simulink model "sampleModel1846"  (R2023a)
settings: Solver=VariableStepAuto  StartTime=0.0  StopTime=10.0  RelTol=1e-3
libraries: hdlsllib x6, simulink x3
settings Model: Creator=user1  LastModifiedBy=user1

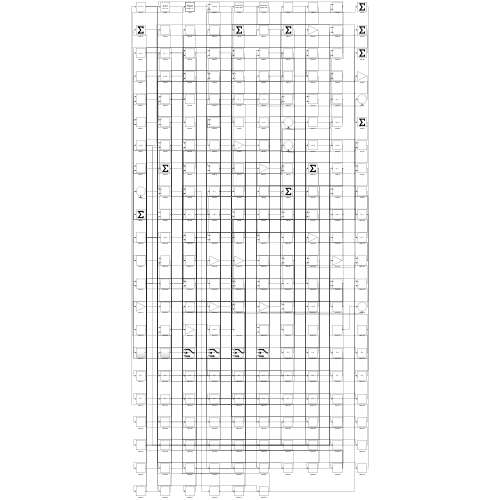
[thumbnail: Simulink's stored preview of the top-level diagram]
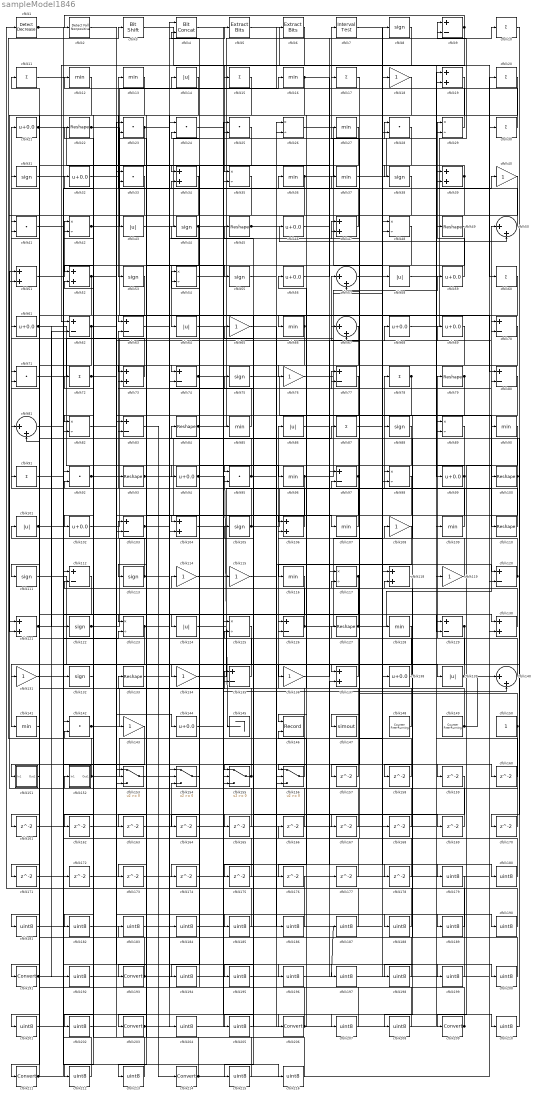
== system sampleModel1846 ==
  cfblk1 : simulink/Logic and Bit Operations/Detect Decrease  vinit=0.0  OutDataTypeStr=boolean
      settings: LibrarySourceBlock=|
      | hdlsllib/Logic and Bit
      | Operations/Detect
      | Decrease
  cfblk{10..11,15,17,20,30,60,72,78,87,91} (11 alike) : Sum  Inputs=+
  cfblk{22,45,49,79,84,93,100,110,127,133} (10 alike) : Reshape
  cfblk{14,43,58,64,86,101,124,139} (8 alike) : Abs  SaturateOnIntegerOverflow=off
  cfblk{21,32,46,56,59,61,68..69,94,99,102,138,144} (13 alike) : Bias  Bias=0.0  SaturateOnIntegerOverflow=off
  cfblk{9,62..63,70,74,77,80,83,97,103,112,120,126,129,135} (15 alike) : Sum  Inputs=+-
  cfblk{19,34,39,47,51..52,73,104,106,118,121,130,137} (13 alike) : Sum
  cfblk{8,31,38,44,53,55,75,88,105,111,113,122,132} (13 alike) : Signum
  cfblk{12..13,16,27,36..37,66,85,90,96,107,109,116,128,141} (15 alike) : MinMax
  cfblk{18,40,65,76,108,114..115,119,131,134,136,143} (12 alike) : Gain
  cfblk{26,29,35,42,48,54,82,89,98,117,123,125} (12 alike) : Product  Inputs=*/  RndMeth=Zero  SaturateOnIntegerOverflow=on
  cfblk{50,57,67,81,140} (5 alike) : Sum  Inputs=|++
  cfblk{23..25,28,33,41,71,92,95,142} (10 alike) : DotProduct  OutDataTypeStr=Inherit: Inherit via internal rule
  cfblk145 : Terminator
  cfblk146 : Record  FileSettingsInternal="{\"entries\":[{\"content\":{\"excelSettings\":{\"content\":{},\"type\":\"Streamout.ExcelSettings\"}},\"type\":\"Streamout.FileSettingStorage\",\"uuid\":\"\"}],\"packageUris\":[\"http:\\/\\/schema.mathworks.com\\/mf0\\/streamout_blocks\\/R2020a\"],\"version\":\"1.0\"}"  Layout=[1 1]  SignalsInternal="{\"entries\":[{\"content\":{\"signals\":[{\"content\":{\"blockPath\":[],\"dimensions\":[1],\"domain\":\"\",\"lineColor\":\"#a2142f\",\"plots\":[1],\"port\":1,\"signalID\":4512,\"signalName\":\"XY Graph:1\"},\"type\":\"RecordBlkView.Signal\",\"uuid\":\"\"},{\"content\":{\"blockPath\":[],\"dimensions\":[1],\"domain\":\"\",\"lineColor\":\"#139fff\",\"plots\":[1],\"port\":2,\"signalID\":4515,\"signalName\":\"XY Graph:2\"},\"type\":\"RecordBlkView.Signal\",\"uuid\":\"\"}]},\"type\":\"RecordBlkView.InputSignals\",\"uuid\":\"\"}],\"packageUris\":[\"http:\\/\\/schema.mathworks.com\\/mf0\\/streamout_blocks\\/R2020a\"],\"version\":\"1.0\"}"  VisualizationBindings="{\"xyplotplugin\":{\"info\":[{\"series\":[{\"bindingParametersList\":[{\"parameter\":\"X-Axis\",\"signalID\":4512,\"signalName\":\"XY Graph:1\"},{\"parameter\":\"Y-Axis\",\"signalID\":4515,\"signalName\":\"XY Graph:2\"}],\"seriesID\":51865}],\"subplotID\":1}]}}"  CompatibilityTag=XY  st=-1
  cfblk147 : ToWorkspace  VariableName=simout  SaveFormat=Timeseries  SampleTime=-1
  cfblk148 : hdlsllib/Sources/Counter Free-Running  NumBits=16  tsamp=-1
  cfblk149 : hdlsllib/Sources/Counter Free-Running  NumBits=16  tsamp=-1
  cfblk150 : Constant  SampleTime=-1
  cfblk151 : Subsystem
      settings: LibrarySourceBlock=|
      | hdlsllib/Ports &
      | Subsystems/Subsystem
  cfblk152 : Subsystem
      settings: LibrarySourceBlock=|
      | hdlsllib/Ports &
      | Subsystems/Subsystem
  cfblk{153..156} (4 alike) : Switch  SaturateOnIntegerOverflow=off  InputSameDT=off
  cfblk{157..178} (22 alike) : Delay  SampleTime=1
  cfblk{179..190,192,194..202,204..205,207..208,210,212..213,215..216} (31 alike) : DataTypeConversion  OutDataTypeStr=uint8  SaturateOnIntegerOverflow=off  RndMeth=Floor
  cfblk{191,193,203,206,209,211,214} (7 alike) : DataTypeConversion  SaturateOnIntegerOverflow=off  RndMeth=Floor
  cfblk2 : hdlsllib/Logic and Bit Operations/Detect Fall Nonpositive  vinit=0  OutDataTypeStr=boolean
  cfblk3 : hdlsllib/Logic and Bit Operations/Bit Shift  mode=Shift Left Logical  N=0
  cfblk4 : hdlsllib/Logic and Bit Operations/Bit Concat  numInputs=2
  cfblk5 : simulink/Logic and Bit Operations/Extract Bits  bitsToExtract=Upper half  numBits=8  bitIdxRange=[0 7]  outScalingMode=Preserve fixed-point scaling
      settings: LibrarySourceBlock=|
      | hdlsllib/Logic and Bit
      | Operations/Extract Bits
  cfblk6 : simulink/Logic and Bit Operations/Extract Bits  bitsToExtract=Upper half  numBits=8  bitIdxRange=[0 7]  outScalingMode=Preserve fixed-point scaling
      settings: LibrarySourceBlock=|
      | hdlsllib/Logic and Bit
      | Operations/Extract Bits
  cfblk7 : hdlsllib/Logic and Bit Operations/Interval Test  IntervalClosedRight=on  uplimit=0.5  IntervalClosedLeft=on  lowlimit=-0.5  OutDataTypeStr=boolean
  wires:
  cfblk29/1 -> cfblk12/1
  cfblk93/1 -> cfblk107/1, cfblk26/1, cfblk173/1
  cfblk121/1 -> cfblk62/2, cfblk123/2, cfblk199/1
  cfblk68/1 -> cfblk9/1
  cfblk127/1 -> cfblk50/1, cfblk45/1
  cfblk8/1 -> cfblk62/1
  cfblk66/1 -> cfblk63/1, cfblk155/1, cfblk123/1
  cfblk156/1 -> cfblk86/1
  cfblk51/1 -> cfblk42/1
  cfblk111/1 -> cfblk136/1
  cfblk99/1 -> cfblk95/1, cfblk155/2
  cfblk76/1 -> cfblk69/1
  cfblk130/1 -> cfblk32/1
  cfblk32/1 -> cfblk16/1
  cfblk10/1 -> cfblk137/1
  cfblk37/1 -> cfblk29/1
  cfblk47/1 -> cfblk13/1
  cfblk5/1 -> cfblk60/1
  cfblk61/1 -> cfblk96/1, cfblk192/1
  cfblk84/1 -> cfblk10/1, cfblk196/1
  cfblk148/1 -> cfblk126/1
  cfblk94/1 -> cfblk145/1, cfblk140/2
  cfblk140/1 -> cfblk79/1
  cfblk9/1 -> cfblk2/1, cfblk15/1
  cfblk45/1 -> cfblk50/2, cfblk37/1
  cfblk4/1 -> cfblk206/1
  cfblk123/1 -> cfblk141/1, cfblk167/1
  cfblk73/1 -> cfblk21/1
  cfblk91/1 -> cfblk36/1
  cfblk34/1 -> cfblk52/1
  cfblk42/1 -> cfblk6/1, cfblk197/1
  cfblk44/1 -> cfblk74/2, cfblk189/1, cfblk213/1
  cfblk69/1 -> cfblk147/1
  cfblk31/1 -> cfblk55/1
  cfblk27/1 -> cfblk82/1
  cfblk152/1(Out1) -> cfblk3/1, cfblk8/1
  cfblk106/1 -> cfblk63/2
  cfblk139/1 -> cfblk56/1, cfblk67/1
  cfblk134/1 -> cfblk70/1
  cfblk96/1 -> cfblk59/1, cfblk174/1
  cfblk92/1 -> cfblk57/1, cfblk94/1
  cfblk26/1 -> cfblk128/1
  cfblk75/1 -> cfblk110/1
  cfblk102/1 -> cfblk46/1
  cfblk56/1 -> cfblk9/2
  cfblk22/1 -> cfblk80/1, cfblk34/1
  cfblk110/1 -> cfblk41/1
  cfblk1/1 -> cfblk130/1, cfblk135/2, cfblk153/2
  cfblk107/1 -> cfblk81/1
  cfblk141/1 -> cfblk11/1
  cfblk50/1 -> cfblk29/2
  cfblk124/1 -> cfblk78/1
  cfblk38/1 -> cfblk76/1
  cfblk151/1(Out1) -> cfblk71/1
  cfblk55/1 -> cfblk40/1
  cfblk72/1 -> cfblk102/1, cfblk68/1
  cfblk18/1 -> cfblk193/1
  cfblk49/1 -> cfblk64/1
  cfblk14/1 -> cfblk53/1
  cfblk125/1 -> cfblk203/1
  cfblk79/1 -> cfblk116/1, cfblk208/1
  cfblk105/1 -> cfblk30/1, cfblk22/1
  cfblk149/1 -> cfblk140/1, cfblk126/2
  cfblk144/1 -> cfblk95/2
  cfblk3/1 -> cfblk99/1
  cfblk113/1 -> cfblk41/2, cfblk77/1
  cfblk6/1 -> cfblk35/1
  cfblk71/1 -> cfblk43/1
  cfblk112/1 -> cfblk211/1
  cfblk20/1 -> cfblk191/1
  cfblk43/1 -> cfblk7/1
  cfblk23/1 -> cfblk5/1, cfblk151/1(In1)
  cfblk132/1 -> cfblk72/1
  cfblk16/1 -> cfblk97/1, cfblk104/2
  cfblk35/1 -> cfblk73/1
  cfblk155/1 -> cfblk103/1, cfblk81/2
  cfblk58/1 -> cfblk100/1
  cfblk154/1 -> cfblk84/1
  cfblk59/1 -> cfblk39/1
  cfblk104/1 -> cfblk98/1
  cfblk64/1 -> cfblk28/1
  cfblk150/1 -> cfblk152/1(In1), cfblk47/2
  cfblk119/1 -> cfblk108/1
  cfblk39/1 -> cfblk38/1, cfblk155/3
  cfblk135/1 -> cfblk93/1
  cfblk153/1 -> cfblk87/1
  cfblk120/1 -> cfblk88/1, cfblk106/2
  cfblk25/1 -> cfblk104/1
  cfblk109/1 -> cfblk27/1
  cfblk138/1 -> cfblk71/2
  cfblk95/1 -> cfblk120/1, cfblk52/2
  cfblk100/1 -> cfblk31/1, cfblk113/1, cfblk170/1
  cfblk62/1 -> cfblk144/1, cfblk111/1
  cfblk142/1 -> cfblk115/1, cfblk135/1
  cfblk88/1 -> cfblk134/1
  cfblk78/1 -> cfblk103/2, cfblk153/3
  cfblk126/1 -> cfblk48/1, cfblk54/1
  cfblk28/1 -> cfblk48/2
  cfblk129/1 -> cfblk146/1, cfblk202/1
  cfblk41/1 -> cfblk39/2
  cfblk122/1 -> cfblk25/2, cfblk85/1
  cfblk52/1 -> cfblk106/1, cfblk161/1
  cfblk90/1 -> cfblk209/1
  cfblk101/1 -> cfblk139/1, cfblk34/2, cfblk210/1, cfblk216/1
  cfblk21/1 -> cfblk117/1, cfblk207/1
  cfblk53/1 -> cfblk82/2
  cfblk85/1 -> cfblk23/2
  cfblk30/1 -> cfblk17/1
  cfblk131/1 -> cfblk132/1
  cfblk137/1 -> cfblk127/1
  cfblk136/1 -> cfblk70/2
  cfblk98/1 -> cfblk154/2
  cfblk36/1 -> cfblk19/1, cfblk121/2
  cfblk12/1 -> cfblk51/2
  cfblk97/1 -> cfblk44/1, cfblk156/2
  cfblk115/1 -> cfblk80/2
  cfblk48/1 -> cfblk156/1
  cfblk74/1 -> cfblk28/2, cfblk124/1, cfblk54/2
  cfblk19/1 -> cfblk66/1
  cfblk116/1 -> cfblk131/1
  cfblk83/1 -> cfblk214/1
  cfblk57/1 -> cfblk129/2
  cfblk103/1 -> cfblk47/1, cfblk77/2, cfblk163/1
  cfblk40/1 -> cfblk74/1
  cfblk117/1 -> cfblk67/2, cfblk212/1
  cfblk17/1 -> cfblk157/1
  cfblk157/1 -> cfblk25/1
  cfblk80/1 -> cfblk158/1
  cfblk158/1 -> cfblk57/2
  cfblk82/1 -> cfblk159/1
  cfblk86/1 -> cfblk160/1
  cfblk160/1 -> cfblk129/1
  cfblk161/1 -> cfblk154/3
  cfblk13/1 -> cfblk162/1
  cfblk162/1 -> cfblk98/2
  cfblk163/1 -> cfblk19/2
  cfblk77/1 -> cfblk164/1
  cfblk81/1 -> cfblk165/1
  cfblk165/1 -> cfblk51/1
  cfblk166/1 -> cfblk154/1
  cfblk167/1 -> cfblk73/2
  cfblk87/1 -> cfblk168/1
  cfblk168/1 -> cfblk42/2
  cfblk54/1 -> cfblk169/1
  cfblk169/1 -> cfblk121/1
  cfblk170/1 -> cfblk117/2
  cfblk15/1 -> cfblk171/1
  cfblk171/1 -> cfblk137/2
  cfblk172/1 -> cfblk35/2
  cfblk173/1 -> cfblk130/2
  cfblk174/1 -> cfblk26/2
  cfblk60/1 -> cfblk175/1
  cfblk175/1 -> cfblk142/1
  cfblk108/1 -> cfblk176/1
  cfblk176/1 -> cfblk1/1
  cfblk177/1 -> cfblk92/2
  cfblk46/1 -> cfblk178/1
  cfblk178/1 -> cfblk97/2
  cfblk114/1 -> cfblk179/1
  cfblk7/1 -> cfblk180/1
  cfblk180/1 -> cfblk114/1
  cfblk33/1 -> cfblk181/1
  cfblk181/1 -> cfblk58/1
  cfblk70/1 -> cfblk182/1
  cfblk182/1 -> cfblk33/1
  cfblk179/1 -> cfblk183/1
  cfblk183/1 -> cfblk33/2
  cfblk133/1 -> cfblk184/1
  cfblk184/1 -> cfblk14/1
  cfblk2/1 -> cfblk185/1
  cfblk185/1 -> cfblk133/1
  cfblk65/1 -> cfblk186/1
  cfblk186/1 -> cfblk23/1
  cfblk187/1 -> cfblk65/1
  cfblk24/1 -> cfblk188/1
  cfblk188/1 -> cfblk92/1
  cfblk189/1 -> cfblk24/1
  cfblk164/1 -> cfblk190/1
  cfblk190/1 -> cfblk24/2
  cfblk191/1 -> cfblk187/1, cfblk119/1, cfblk138/1
  cfblk192/1 -> cfblk20/1
  cfblk193/1 -> cfblk49/1, cfblk61/1
  cfblk128/1 -> cfblk194/1
  cfblk194/1 -> cfblk18/1
  cfblk89/1 -> cfblk195/1
  cfblk195/1 -> cfblk177/1
  cfblk196/1 -> cfblk89/1
  cfblk197/1 -> cfblk89/2
  cfblk118/1 -> cfblk198/1
  cfblk198/1 -> cfblk166/1
  cfblk199/1 -> cfblk118/1
  cfblk11/1 -> cfblk200/1
  cfblk200/1 -> cfblk118/2
  cfblk143/1 -> cfblk201/1
  cfblk201/1 -> cfblk122/1
  cfblk202/1 -> cfblk143/1
  cfblk203/1 -> cfblk156/3, cfblk109/1
  cfblk63/1 -> cfblk204/1
  cfblk204/1 -> cfblk125/1
  cfblk159/1 -> cfblk205/1
  cfblk205/1 -> cfblk125/2
  cfblk206/1 -> cfblk146/2, cfblk142/2
  cfblk207/1 -> cfblk4/1
  cfblk208/1 -> cfblk4/2
  cfblk209/1 -> cfblk75/1, cfblk91/1, cfblk105/1
  cfblk210/1 -> cfblk90/1
  cfblk211/1 -> cfblk172/1, cfblk101/1
  cfblk212/1 -> cfblk112/1
  cfblk213/1 -> cfblk112/2
  cfblk214/1 -> cfblk153/1, cfblk120/2
  cfblk67/1 -> cfblk215/1
  cfblk215/1 -> cfblk83/1
  cfblk216/1 -> cfblk83/2

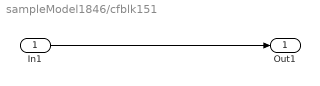
== system sampleModel1846/cfblk151 ==
  In1 : Inport
  Out1 : Outport
  wires:
  In1/1 -> Out1/1

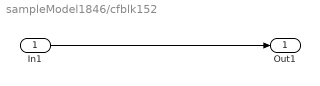
== system sampleModel1846/cfblk152 ==
  In1 : Inport
  Out1 : Outport
  wires:
  In1/1 -> Out1/1
